simulink model "testmodele1"  (R2021a)
settings: Solver=FixedStepAuto  StartTime=0.0  StopTime=1.5  FixedStep=0.001  RelTol=1e-3
undefined symbols (not defined in the file): B, C, Crr, D, E, f, h, I_z, J, K_a, K_phi, K_r, L, L_ar, L_av, M, p, R, Res, S_x, S_y, W
libraries: slpidlib x8
settings Model: Creator=TP-EEA  LastModifiedBy=TP-EEA

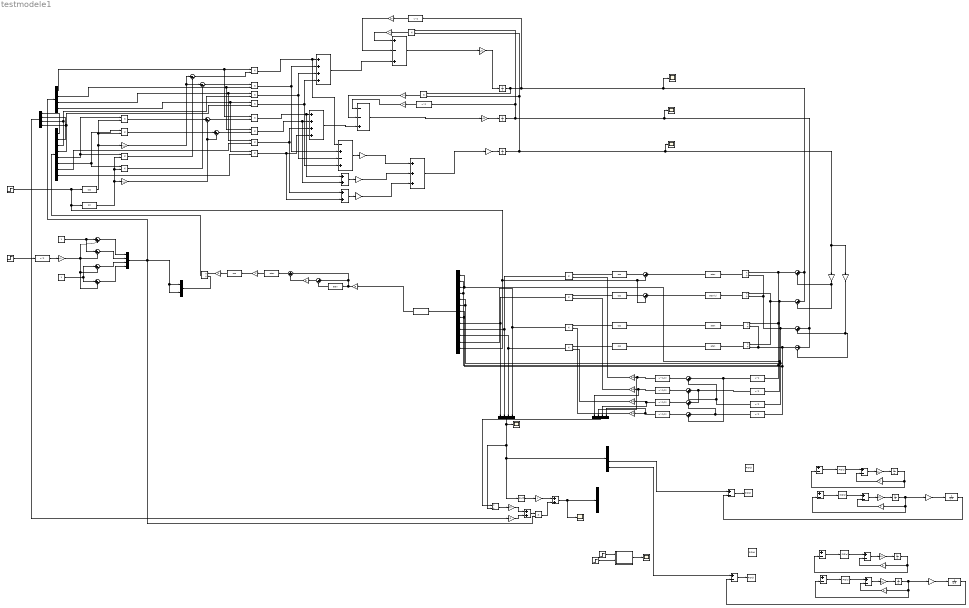
== system testmodele1 ==
  note: Onduleur
  note: Moteur+commande
  note: vecteur des omega_i*
  note: Entrées
  note: Eq (1)
  note: 1er terme (1)
  note: µ1
  note: Calcul des µ_i
  note: Calcul des lambda_i et lambda_v_i
  note: Calcul des réactions normales pour chaque roue
  note: N°12
  note: Calcul de la vitesse de rotation pour chaque roue
  note: Calcul des vitesses à chaque roue
  note: u2=u4
  note: Angle Alpha pour chaque roue
  note: u+wrW/2
  note: V^2
  note: delta_N
  note: u-wrW/2
  note: v-L_av*wr
  note: v+L_av*wr
  note: u1=u3
  note: v1=v2
  note: v3=v4
  note: (u2=u4)^2
  note: (u1=u3)^2
  note: (v1=v2)^2
  note: (v3=v4)^2
  note: N°34
  note: µ2
  note: µ3
  note: µ4
  note: µv4
  note: µv2
  note: µv1
  note: µv3
  note: N1
  note: N2
  note: N3
  note: N4
  note: Kr*cos(Beta)
  note: µv2*cos(Beta)
  note: µv1*cos(Beta)
  note: µv1*sin(Beta)
  note: µv2*sin(Beta)
  note: Kr*sin(Beta)
  note: 2eme terme (1)
  note: 3eme terme (1)
  note: 4eme terme (1)
  note: 1er terme (2)
  note: 2eme terme (2)
  note: 3eme terme (2)
  note: 4eme terme (2)
  note: Eq (2)
  note: Eq (3)
  note: vecteur des V_i
  note: Calcul des couples moteurs
  note: Moteur+commande
  note: Onduleur
  Add : Sum  Inputs=++++
  Add1 : Sum  Inputs=++++
  Add{10..19} (10 alike) : Sum  Inputs=+-
  Add2 : Sum  Inputs=+-+
  Add3 : Sum  Inputs=--+
  Add{4,6,8..9} (4 alike) : Sum
  Add5 : Sum  Inputs=-+-+
  Add7 : Sum  Inputs=+++
  Constant : Constant
  Constant1 : Constant
  Demux1 : Demux  Outputs=8
  Demux2 : Demux
  Demux3 : Demux
  Demux4 : Demux
  Derivative : Derivative
  Divide{,1..5} (6 alike) : Product  Inputs=*/
  Gain : Gain  Gain=1/M
  Gain1 : Gain  Gain=1/M
  Gain10 : Gain  Gain=B
  Gain11 : Gain  Gain=E
  Gain12 : Gain  Gain=C
  Gain13 : Gain  Gain=D
  Gain14 : Gain  Gain=K_r
  Gain15 : Gain  Gain=K_r
  Gain16 : Gain  Gain=M
  Gain17 : Gain  Gain=K_a*S_x
  Gain18 : Gain  Gain=M
  Gain19 : Gain  Gain=K_a*S_y
  Gain2 : Gain  Gain=1/I_z
  Gain20 : Gain  Gain=L_av
  Gain21 : Gain  Gain=W/2
  Gain22 : Gain  Gain=-L_ar
  Gain{23,27,29,32,34} (5 alike) : Gain  Gain=R
  Gain24 : Gain  Gain=Crr
  Gain25 : Gain  Gain=J
  Gain{26,28,31,33} (4 alike) : Gain  Gain=1/L
  Gain3 : Gain  Gain=M*h/(2*R*W)
  Gain30 : Gain  Gain=K_phi
  Gain35 : Gain  Gain=K_phi
  Gain4 : Gain  Gain=W/2
  Gain5 : Gain  Gain=L_av
  Gain{6..9} (4 alike) : Gain  Gain=1/R
  Integrator : Integrator  InitialCondition=0.001
  Integrator1 : Integrator  InitialCondition=0.001
  Integrator2 : Integrator  InitialCondition=0.001
  Integrator{3..6} (4 alike) : Integrator
  Interpreted MATLAB Function : MATLABFcn
  Interpreted MATLAB Function{1,7..10,21} (6 alike) : MATLABFcn  MATLABFcn=cos
  Interpreted MATLAB Function{2,11..14,23..24} (7 alike) : MATLABFcn  MATLABFcn=u^2
  Interpreted MATLAB Function{15..18} (4 alike) : MATLABFcn  MATLABFcn=u^(1/2)
  Interpreted MATLAB Function{3,5..6,19..20} (5 alike) : MATLABFcn  MATLABFcn=atan
  Interpreted MATLAB Function22 : MATLABFcn  MATLABFcn=calcul_lambda
  Interpreted MATLAB Function4 : MATLABFcn  MATLABFcn=atan(u)
  MSAP : Subsystem
  Mux : Mux  Inputs=13
  Mux{1,3..5} (4 alike) : Mux
  Mux2 : Mux  Inputs=2
  PID Controller{,1..7} (8 alike) : slpidlib/PID Controller  Controller=PID  Form=Parallel  TimeDomain=Continuous-time  UseExternalTs=off  SampleTime=-1  IntegratorMethod=Forward Euler  FilterMethod=Forward Euler  ControllerParametersSource=internal  P=1  I=1  D=0  UseFilter=on  N=100  TunerSelectOption=Transfer Function Based (PID Tuner App)  InitialConditionSource=internal  InitialConditionForIntegrator=0  InitialConditionForFilter=0  DifferentiatorICPrevScaledInput=0  ExternalReset=none  TrackingMode=off  Kt=1  LimitOutput=off  SatLimitsSource=internal  UpperSaturationLimit=inf  LowerSaturationLimit=-inf  LinearizeAsGain=on  AntiWindupMode=none  Kb=1  POutMin=[]  POutMax=[]  IOutMin=[]  IOutMax=[]  DOutMin=[]  DOutMax=[]  NOutMin=[]  NOutMax=[]  SumOutMin=[]  SumOutMax=[]  SaturationOutMin=[]  SaturationOutMax=[]  PParamMin=[]  PParamMax=[]  IParamMin=[]  IParamMax=[]  DParamMin=[]  DParamMax=[]  NParamMin=[]  NParamMax=[]  KbParamMin=[]  KbParamMax=[]  KtParamMin=[]  KtParamMax=[]  KbOutMin=[]  KbOutMax=[]  KtOutMin=[]  KtOutMax=[]  IntegratorOutMin=[]  IntegratorOutMax=[]  FilterOutMin=[]  FilterOutMax=[]  SumI1OutMin=[]  SumI1OutMax=[]  SumI2OutMin=[]  SumI2OutMax=[]  SumI3OutMin=[]  SumI3OutMax=[]  SumI4OutMin=[]  SumI4OutMax=[]  SumDOutMin=[]  SumDOutMax=[]  DifferentiatorOutMin=[]  DifferentiatorOutMax=[]  FilterDiffOutCoefMin=[]  FilterDiffOutCoefMax=[]  ReciprocalOutMin=[]  ReciprocalOutMax=[]  SumDenOutMin=[]  SumDenOutMax=[]  SumNumOutMin=[]  SumNumOutMax=[]  DivideOutMin=[]  DivideOutMax=[]  UdiffTsProdOutMin=[]  UdiffTsProdOutMax=[]  NTsProdOutMin=[]  NTsProdOutMax=[]  UintegralTsProdOutMin=[]  UintegralTsProdOutMax=[]  UngainTsProdOutMin=[]  UngainTsProdOutMax=[]  IntegratorContinuousStateAttributes=''  IntegratorStateMustResolveToSignalObject=off  IntegratorRTWStateStorageClass=Auto  FilterContinuousStateAttributes=''  FilterStateMustResolveToSignalObject=off  FilterRTWStateStorageClass=Auto  ParallelPVariant=InternalParameters  IdealPVariant=Disabled  IVariant=InternalParameters  DVariant=InternalParameters  IntegratorVariant=Continuous  SatVariant=Disabled  AWVariant=Passthrough  PCopyVariant=Disabled  TRVariant=Disabled  FdbkBlocksVariant=Forward  IdealPFdbkVariant=Disabled  SatFdbkVariant=Disabled  DerivativeFilterVariant=ContFilter  NVariant=InternalParameters  NCopyVariant=Disabled  FilterICVariant=InternalICsFilter  IntegratorICVariant=InternalICs  ExternalResetVariant=Disabled  TRSumVariant=Passthrough  SumFdbkVariant=Disabled  SumVariant=Sum_PID  TsampFilterVariant=InternalTs  TsampNgainVariant=Passthrough  TsampIntegralVariant=Passthrough  ExternalSaturationOutDataTypeStr=Inherit: Same as second input
  Product{1..19} (19 alike) : Product
  Scope{,1..5} (6 alike) : Scope
  Step : Step  Time=0  Before=0.1  After=0.2  SampleTime=0
  Step1 : Step  Time=0  SampleTime=0
  Step2 : Step  Time=0  SampleTime=0
  Step3 : Step  Time=0  SampleTime=0
  Sum{,2,6..11} (8 alike) : Sum  Inputs=|++
  Sum{1,3..5,12..15,18..19} (10 alike) : Sum  Inputs=|+-
  Sum16 : Sum  Inputs=|--
  Sum17 : Sum  Inputs=|--
  Transfer Fcn1 : TransferFcn  Denominator=[J f]
  Transfer Fcn2 : TransferFcn  Denominator=[J f]
  wires:
  Step/1 -> Interpreted MATLAB Function/1, Sum4/2, Sum5/2, Mux/13, Interpreted MATLAB Function1/1  "angle Beta"
  Gain2/1 -> Integrator1/1
  Gain1/1 -> Integrator2/1
  Gain/1 -> Integrator/1
  Step1/1 -> Interpreted MATLAB Function2/1  "V*"
  Interpreted MATLAB Function2/1 -> Gain3/1
  Integrator/1 -> Product18/1, Interpreted MATLAB Function23/1, Scope/1, Sum1/1, Sum/1  "u"
  Integrator2/1 -> Product17/1, Interpreted MATLAB Function24/1, Scope1/1, Sum3/1, Sum2/1  "v"
  Integrator1/1 -> Product18/2, Product17/2, Scope2/1, Gain5/1, Gain4/1  "omega_r"
  Gain4/1 -> Sum/2, Sum1/2
  Gain5/1 -> Sum3/2, Sum2/2
  Sum1/1 -> Interpreted MATLAB Function12/1, Mux/1, Mux/3, Divide/1, Divide2/1
  Sum2/1 -> Interpreted MATLAB Function13/1, Mux/5, Mux/6, Divide/2, Divide1/2
  Sum/1 -> Divide1/1, Interpreted MATLAB Function11/1, Mux/2, Mux/4, Divide3/1
  Sum3/1 -> Interpreted MATLAB Function14/1, Mux/7, Mux/8, Divide2/2, Divide3/2
  Divide1/1 -> Interpreted MATLAB Function3/1
  Divide/1 -> Interpreted MATLAB Function4/1
  Divide3/1 -> Interpreted MATLAB Function5/1
  Divide2/1 -> Interpreted MATLAB Function6/1
  Interpreted MATLAB Function3/1 -> Sum4/1  "alpha2"
  Interpreted MATLAB Function4/1 -> Sum5/1  "alpha1"
  Interpreted MATLAB Function6/1 -> Interpreted MATLAB Function10/1  "alpha3"
  Interpreted MATLAB Function5/1 -> Interpreted MATLAB Function9/1  "alpha4"
  Sum5/1 -> Interpreted MATLAB Function8/1
  Sum4/1 -> Interpreted MATLAB Function7/1
  Interpreted MATLAB Function12/1 -> Sum8/1, Sum7/1
  Interpreted MATLAB Function13/1 -> Sum7/2, Sum6/2
  Interpreted MATLAB Function11/1 -> Sum9/2, Sum6/1
  Interpreted MATLAB Function14/1 -> Sum9/1, Sum8/2
  Sum9/1 -> Interpreted MATLAB Function18/1
  Sum8/1 -> Interpreted MATLAB Function17/1
  Sum7/1 -> Interpreted MATLAB Function16/1
  Sum6/1 -> Interpreted MATLAB Function15/1
  Interpreted MATLAB Function15/1 -> Gain6/1, Mux5/2  "V2"
  Interpreted MATLAB Function16/1 -> Gain7/1, Mux5/1  "V1"
  Interpreted MATLAB Function17/1 -> Gain8/1, Mux5/3  "V3"
  Interpreted MATLAB Function18/1 -> Gain9/1, Mux5/4  "V4"
  Interpreted MATLAB Function7/1 -> Product4/1
  Interpreted MATLAB Function8/1 -> Product5/1
  Interpreted MATLAB Function9/1 -> Product6/1
  Interpreted MATLAB Function10/1 -> Product7/1
  Gain6/1 -> Product4/2
  Gain7/1 -> Product5/2
  Gain9/1 -> Product6/2
  Gain8/1 -> Product7/2
  Constant1/1 -> Sum13/1, Sum10/1
  Gain3/1 -> Sum13/2, Sum12/2, Sum11/2, Sum10/2
  Constant/1 -> Sum12/1, Sum11/1
  Gain10/1 -> Sum15/1, Sum14/1, Interpreted MATLAB Function19/1
  Interpreted MATLAB Function19/1 -> Sum14/2
  Sum14/1 -> Gain11/1
  Gain11/1 -> Sum15/2
  Sum15/1 -> Interpreted MATLAB Function20/1
  Interpreted MATLAB Function20/1 -> Gain12/1
  Gain12/1 -> Interpreted MATLAB Function21/1
  Interpreted MATLAB Function21/1 -> Gain13/1
  Gain13/1 -> Divide4/1
  Product5/1 -> Mux4/1, Mux/9  "omega1"
  Product4/1 -> Mux4/2, Mux/10  "omega2"
  Product7/1 -> Mux/11, Mux4/3  "omega3"
  Product6/1 -> Mux/12, Mux4/4  "omega4"
  Mux/1 -> Interpreted MATLAB Function22/1
  Sum10/1 -> Mux1/1  "N1"
  Sum13/1 -> Mux1/2  "N2"
  Sum12/1 -> Mux1/3  "N3"
  Sum11/1 -> Mux1/4  "N4"
  Mux1/1 -> Product19/2, Mux2/2, Mux2/1, Demux2/1  "vecteur des N_i"
  Mux2/1 -> Divide4/2
  Interpreted MATLAB Function22/1 -> Gain10/1  "Vecteur des lambda_i et lambda_v_i"
  Divide4/1 -> Demux1/1  "Vecteur des µ_i et µ_v_i"
  Interpreted MATLAB Function1/1 -> Product1/2, Product2/2, Gain14/1  "cos(Beta)"
  Demux1/5 -> Product1/1, Product8/1
  Demux1/6 -> Product3/1, Product2/1
  Interpreted MATLAB Function/1 -> Product3/2, Product8/2, Gain15/1  "sin(Beta)"
  Gain14/1 -> Sum17/1, Sum16/1
  Product8/1 -> Sum16/2
  Demux2/1 -> Product13/1, Product9/1
  Sum16/1 -> Product9/2
  Product3/1 -> Sum17/2
  Demux2/2 -> Product10/2, Product14/1
  Sum17/1 -> Product10/1
  Demux2/3 -> Product15/1, Product12/1
  Demux1/3 -> Mux3/3, Product12/2
  Demux2/4 -> Product16/1, Product11/1
  Demux1/4 -> Product11/2, Mux3/4
  Product1/1 -> Sum18/1
  Gain15/1 -> Sum19/2, Sum18/2
  Sum18/1 -> Product13/2
  Product2/1 -> Sum19/1
  Sum19/1 -> Product14/2
  Demux1/7 -> Product15/2
  Demux1/8 -> Product16/2
  Product9/1 -> Add5/1, Add/1
  Product10/1 -> Add/2, Add5/2
  Product12/1 -> Add/3, Add5/3
  Product11/1 -> Add5/4, Add/4
  Product13/1 -> Add4/1, Add1/1
  Product14/1 -> Add4/2, Add1/2
  Product15/1 -> Add6/1, Add1/3
  Product16/1 -> Add6/2, Add1/4
  Product17/1 -> Gain16/1
  Interpreted MATLAB Function23/1 -> Gain17/1
  Add/1 -> Add2/3
  Gain16/1 -> Add2/1
  Gain17/1 -> Add2/2
  Add2/1 -> Gain/1
  Product18/1 -> Gain18/1
  Interpreted MATLAB Function24/1 -> Gain19/1
  Add1/1 -> Add3/3
  Gain19/1 -> Add3/1
  Gain18/1 -> Add3/2
  Add3/1 -> Gain1/1
  Add4/1 -> Gain20/1
  Add5/1 -> Gain21/1
  Add6/1 -> Gain22/1
  Gain21/1 -> Add7/1
  Gain20/1 -> Add7/2
  Gain22/1 -> Add7/3
  Add7/1 -> Gain2/1
  Demux1/1 -> Mux3/1
  Demux1/2 -> Mux3/2
  Mux4/1 -> Divide5/2, Derivative/1, Demux4/1, Scope3/1
  Mux5/1 -> Divide5/1
  Derivative/1 -> Gain25/1
  Divide5/1 -> Gain24/1
  Mux3/1 -> Gain23/1  "vecteur des µ_i"
  Gain24/1 -> Add8/1
  Gain23/1 -> Add8/2
  Add8/1 -> Product19/1
  Gain25/1 -> Add9/1
  Product19/1 -> Add9/2
  Add9/1 -> Demux3/1, Scope4/1  "Vecteur des couples moteurs*"
  Step2/1 -> MSAP/1(v_q)  "v_q"
  Step3/1 -> MSAP/2(v_d)  "v_d"
  MSAP/1(omega) -> Scope5/1
  Gain26/1 -> Integrator3/1
  Gain27/1 -> Add12/2
  Integrator3/1 -> Gain30/1, Gain27/1, Add10/2  "i_q"
  PID Controller/1 -> Add12/1
  Add10/1 -> PID Controller/1
  Add12/1 -> Gain26/1
  ? -> Add10/1
  PID Controller1/1 -> Add13/1
  Add11/1 -> PID Controller1/1
  Add13/1 -> Gain28/1
  Gain29/1 -> Add13/2
  Gain28/1 -> Integrator4/1
  ? -> Add11/1
  Integrator4/1 -> Gain29/1, Add11/2  "i_d"
  Gain30/1 -> Transfer Fcn2/1  "T_e"
  Add14/1 -> PID Controller3/1
  Transfer Fcn2/1 -> Add14/2  "omega"
  Demux4/3 -> Add14/1  "omega3*"
  PID Controller4/1 -> Add17/1
  ? -> Add15/1
  ? -> Add16/1
  Gain33/1 -> Integrator6/1
  Gain34/1 -> Add18/2
  Add18/1 -> Gain33/1
  Add16/1 -> PID Controller5/1
  PID Controller5/1 -> Add18/1
  Add15/1 -> PID Controller4/1
  Add17/1 -> Gain31/1
  Gain32/1 -> Add17/2
  Gain31/1 -> Integrator5/1
  Integrator6/1 -> Gain34/1, Add16/2  "i_d"
  Transfer Fcn1/1 -> Add19/2  "omega"
  Add19/1 -> PID Controller7/1
  Gain35/1 -> Transfer Fcn1/1  "T_e"
  Demux4/4 -> Add19/1  "omega3*"
  Integrator5/1 -> Gain35/1, Gain32/1, Add15/2  "i_q"

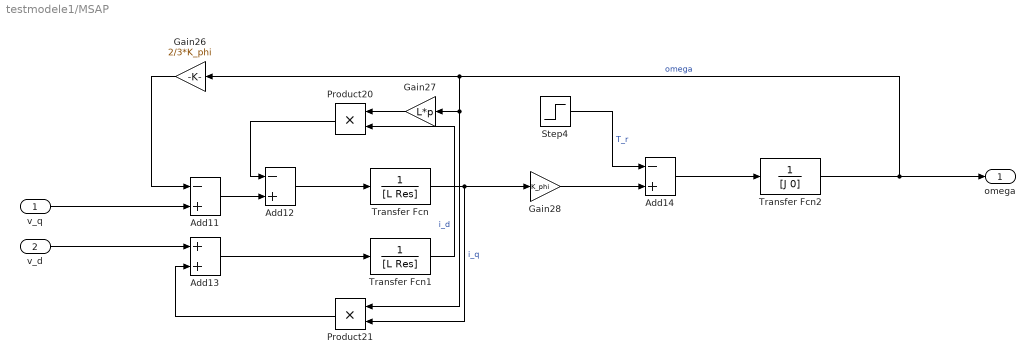
== system testmodele1/MSAP ==
  v_q : Inport
  v_d : Inport  Port=2
  Add11 : Sum  Inputs=-+
  Add12 : Sum  Inputs=-+
  Add13 : Sum
  Add14 : Sum  Inputs=-+
  Gain26 : Gain  Gain=2/3*K_phi
  Gain27 : Gain  Gain=L*p
  Gain28 : Gain  Gain=K_phi
  Product20 : Product
  Product21 : Product
  Step4 : Step  Time=0  SampleTime=0
  Transfer Fcn : TransferFcn  Denominator=[L Res]
  Transfer Fcn1 : TransferFcn  Denominator=[L Res]
  Transfer Fcn2 : TransferFcn  Denominator=[J 0]
  omega : Outport
  wires:
  Gain26/1 -> Add11/1
  Product21/1 -> Add13/2
  Add14/1 -> Transfer Fcn2/1
  Transfer Fcn1/1 -> Product20/2  "i_d"
  Transfer Fcn2/1 -> omega/1, Product21/1, Gain27/1, Gain26/1  "omega"
  Gain27/1 -> Product20/1
  Transfer Fcn/1 -> Product21/2, Gain28/1  "i_q"
  Add12/1 -> Transfer Fcn/1
  Add11/1 -> Add12/2
  Gain28/1 -> Add14/2
  Product20/1 -> Add12/1
  Add13/1 -> Transfer Fcn1/1
  Step4/1 -> Add14/1  "T_r"
  v_d/1 -> Add13/1
  v_q/1 -> Add11/2
